simulink model "T3"  (R2018a)
settings: Solver=VariableStepAuto  StartTime=0.0  StopTime=50  RelTol=1e-3
values from neighbouring files (symbols this model uses):
  Ian = 2.2    [Parameter_DCM_Modified1.m]
  J = 9.5257e-2    (= 0.095257)    [Parameter_DCM_Modified1.m]
  La = 0.1677    [Parameter_DCM_Modified1.m]
  Lf = 0.2    [Parameter_DCM_Modified1.m]
  Ra = 25    [Parameter_DCM_Modified1.m]
  Rf = 590    [Parameter_DCM_Modified1.m]
  Tl = 3    [Parameter_DCM_Modified1.m]
  Van = 220    [Parameter_DCM_Modified1.m]
  Vfn = 220    [Parameter_DCM_Modified1.m]
  wn = (2*pi*Nn)/60    (= 247.138622082)    [Parameter_DCM_Modified1.m]
settings Model: Creator=663tu  LastModifiedBy=663tu

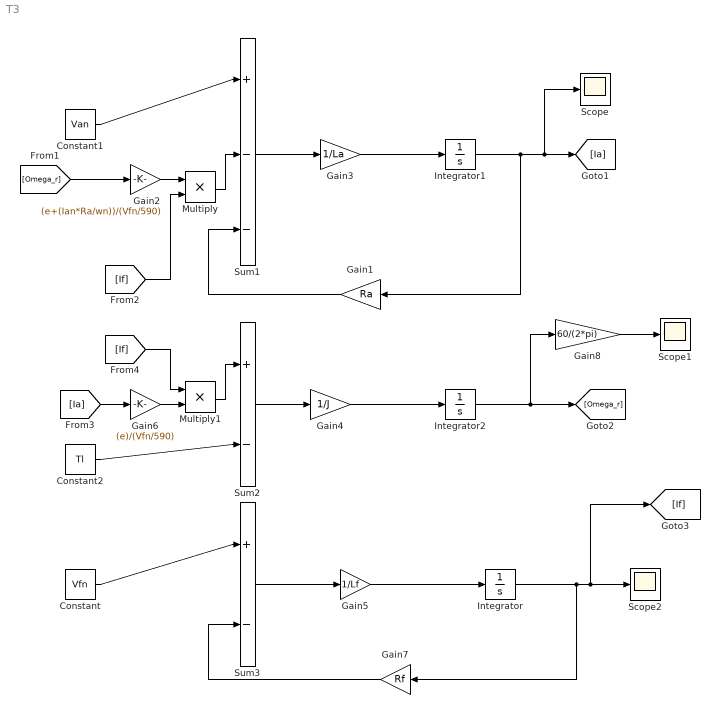
== system T3 ==
  Constant : Constant  Value=Vfn
  Constant1 : Constant  Value=Van
  Constant2 : Constant  Value=Tl
  Gain1 : Gain  Gain=Ra
  Gain2 : Gain  Gain=(e+(Ian*Ra/wn))/(Vfn/590)
  Gain3 : Gain  Gain=1/La
  Gain4 : Gain  Gain=1/J
  Gain5 : Gain  Gain=1/Lf
  Gain6 : Gain  Gain=(e)/(Vfn/590)
  Gain7 : Gain  Gain=Rf
  Gain8 : Gain  Gain=60/(2*pi)
  Integrator : Integrator
  Integrator1 : Integrator
  Integrator2 : Integrator
  Multiply : Product
  Multiply1 : Product
  Scope : Scope
  Scope1 : Scope
  Scope2 : Scope
  Sum1 : Sum  Inputs=|+--
  Sum2 : Sum  Inputs=|+-
  Sum3 : Sum  Inputs=|+-
  wires:
  Gain3/1 -> Integrator1/1
  Gain8/1 -> Scope1/1
  Constant2/1 -> Sum2/2
  Constant1/1 -> Sum1/1
  Gain4/1 -> Integrator2/1
  Gain1/1 -> Sum1/3
  Gain5/1 -> Integrator/1
  Gain7/1 -> Sum3/2
  Sum1/1 -> Gain3/1
  Integrator2/1 -> Gain8/1, [Omega_r]
  [Ia] -> Gain6/1
  Sum3/1 -> Gain5/1
  Constant/1 -> Sum3/1
  Integrator1/1 -> Gain1/1, Scope/1, [Ia]
  Sum2/1 -> Gain4/1
  [Omega_r] -> Gain2/1
  Integrator/1 -> Gain7/1, [If], Scope2/1
  Gain2/1 -> Multiply/1
  Multiply/1 -> Sum1/2
  [If] -> Multiply/2
  Gain6/1 -> Multiply1/2
  Multiply1/1 -> Sum2/1
  [If] -> Multiply1/1
